simulink model "SimulinkPacer"  (R2022a)
settings: Solver=FixedStepAuto  StartTime=0.0  StopTime=10.0  FixedStep=1e-3  RelTol=1e-3  EnableMultiTasking=on
undefined symbols (not defined in the file): D0, D1, D10, D11, D12, D13, D2, D3, D4, D5, D6, D7, D8, D9, PTA0, PTA1, PTA2, PTB23, PTB9, PTC16, PTC17, PTC2, PTC3, PTC4, PTD0, PTD1, PTD2, PTD3
libraries: frdmk64flib x17
settings Model: ExtModeTrigDuration=5  Creator=sabri  LastModifiedBy=Tim
settings SolverCC: AlgebraicLoopSolver=TrustRegion
settings OptimizationCC: EnhancedBackFolding=on  PassReuseOutputArgsAs=Individual arguments  ZeroExternalMemoryAtStartup=off  ZeroInternalMemoryAtStartup=off  MaxStackSize=64  OptimizeBlockOrder=speed  DifferentSizesBufferReuse=on  OptimizationCustomize=off  EfficientTunableParamExpr=on
settings DebuggingCC: ParameterTunabilityLossMsg=error  UnconnectedInputMsg=warning  UnconnectedOutputMsg=warning  UnconnectedLineMsg=warning  SFMachineParentedDataDiag=warning
settings HardwareCC: ProdBitPerPointer=32  ProdBitPerSizeT=32  ProdBitPerPtrDiffT=32  ProdLargestAtomicInteger=Long  ProdLargestAtomicFloat=Double  ProdWordSize=32  ProdHWDeviceType=ARM Compatible->ARM Cortex
settings SFSimCC: MATLABDynamicMemAlloc=off
settings RTWCC: SystemTargetFile=ert.tlc  HardwareBoard=NXP FRDM-K64F  TLCOptions="-aInlineSetEventsForThisBaseRateFcn=TLC_FALSE -aSuppressMultiTaskScheduler=TLC_FALSE  -aRateBasedStepFcn=0"  TemplateMakefile=ert_default_tmf  Toolchain=GNU Tools for ARM Embedded Processors
settings CodeAppCC: ForceParamTrailComments=on  IgnoreCustomStorageClasses=off  OperatorAnnotations=on  SimulinkDataObjDesc=on  SFDataObjDesc=on  InsertBlockDesc=on

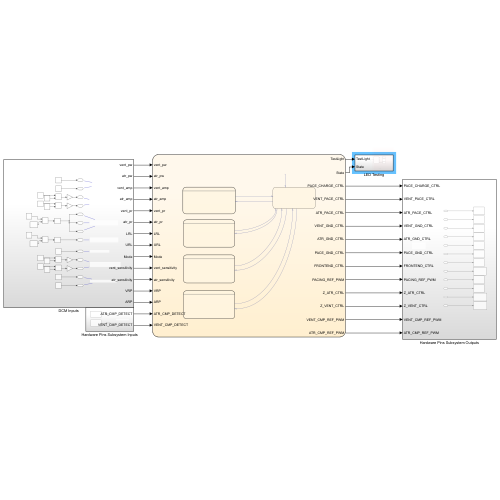
[thumbnail: Simulink's stored preview of the top-level diagram]
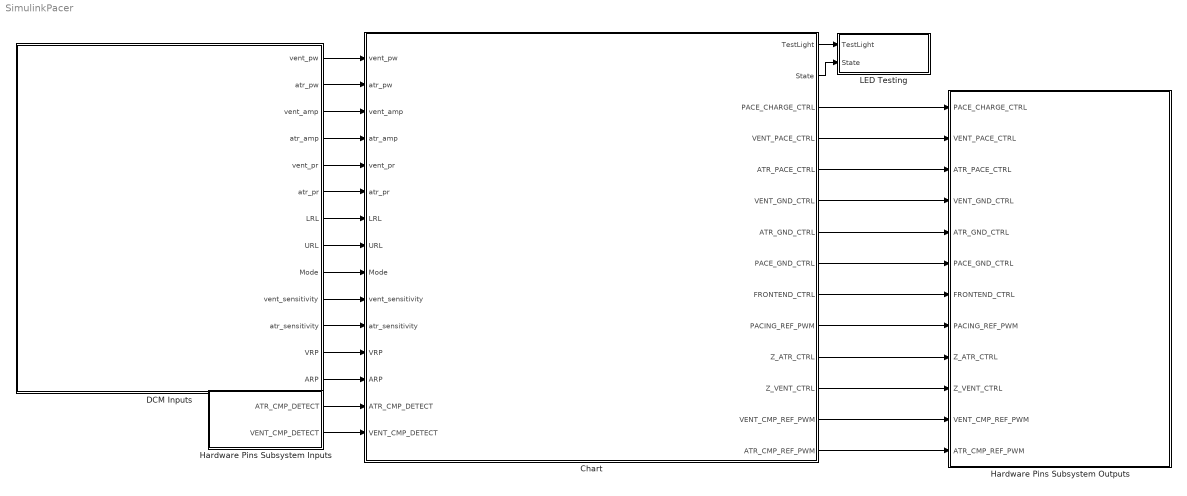
== system SimulinkPacer ==
  Chart : Stateflow chart  TreatAsAtomicUnit=on
      settings: PortSchema="{\"entries\":[{\"content\":{\"sides\":[{\"content\":{\"connectorIds\":[\"In1\",\"In2\",\"In3\",\"In4\",\"In5\",\"In8\",\"In6\",\"In7\",\"In9\",\"In13\",\"In15\",\"In12\",\"In14\",\"In10\",\"In11\"]},\"type\":\"ConnectorPlacement.EquallySpacedRectSide\",\"uuid\":\"c98da620-bdff-4f08-8425-4ebbcd1bf391\"},{\"content\":{\"connectorIds\":[\"Out14\",\"Out1\",\"Out2\",\"Out3\",\"Out4\",\"Out5\",\"Out6\",\"Out7\",\"Out8\",\"Out9\",\"Out10\",\"Out11\",\"Out12\",\"Out13\"],\"side\":\"RIGHT\"},\"type\":\"ConnectorPlacement.EquallySpacedRectSide\",\"uuid\":\"56adc0a6-f124-4dd5-8d25-ce86442aaf81\"},{\"content\":{\"connectorIds\":[],\"side\":\"TOP\"},\"type\":\"ConnectorPlacement.EquallySpacedRectSide\",\"uuid\":\"2a0b7820-84a3-4d69-9bc9-487093068e4c\"}]},\"type\":\"ConnectorPlacement.EquallySpacedConnector\",\"uuid\":\"3fd3921a-48fb-429d-b48c-ef226cae10fe\"}],\"packageUris\":[\"http://schema.mathworks.com/mf0/Connector/R2020b\"],\"version\":\"1.0\"}"
  DCM Inputs : Subsystem
  Hardware Pins Subsystem Inputs : Subsystem
  Hardware Pins Subsystem Outputs : Subsystem
  LED Testing : Subsystem
  wires:
  Chart/2(PACE_CHARGE_CTRL) -> Hardware Pins Subsystem Outputs/1(PACE_CHARGE_CTRL)
  Chart/3(VENT_PACE_CTRL) -> Hardware Pins Subsystem Outputs/2(VENT_PACE_CTRL)
  Chart/4(ATR_PACE_CTRL) -> Hardware Pins Subsystem Outputs/3(ATR_PACE_CTRL)
  Chart/5(VENT_GND_CTRL) -> Hardware Pins Subsystem Outputs/4(VENT_GND_CTRL)
  Chart/6(ATR_GND_CTRL) -> Hardware Pins Subsystem Outputs/5(ATR_GND_CTRL)
  Chart/7(PACE_GND_CTRL) -> Hardware Pins Subsystem Outputs/6(PACE_GND_CTRL)
  Chart/8(FRONTEND_CTRL) -> Hardware Pins Subsystem Outputs/7(FRONTEND_CTRL)
  Chart/9(PACING_REF_PWM) -> Hardware Pins Subsystem Outputs/8(PACING_REF_PWM)
  Chart/10(Z_ATR_CTRL) -> Hardware Pins Subsystem Outputs/9(Z_ATR_CTRL)
  Chart/11(Z_VENT_CTRL) -> Hardware Pins Subsystem Outputs/10(Z_VENT_CTRL)
  DCM Inputs/1(vent_pw) -> Chart/1(vent_pw)
  DCM Inputs/2(atr_pw) -> Chart/2(atr_pw)
  DCM Inputs/3(vent_amp) -> Chart/3(vent_amp)
  DCM Inputs/4(atr_amp) -> Chart/4(atr_amp)
  DCM Inputs/5(vent_pr) -> Chart/5(vent_pr)
  DCM Inputs/6(atr_pr) -> Chart/8(atr_pr)
  DCM Inputs/9(Mode) -> Chart/9(Mode)
  Hardware Pins Subsystem Inputs/2(VENT_CMP_DETECT) -> Chart/11(VENT_CMP_DETECT)
  Hardware Pins Subsystem Inputs/1(ATR_CMP_DETECT) -> Chart/10(ATR_CMP_DETECT)
  DCM Inputs/7(LRL) -> Chart/6(LRL)
  DCM Inputs/8(URL) -> Chart/7(URL)
  DCM Inputs/12(VRP) -> Chart/12(VRP)
  DCM Inputs/13(ARP) -> Chart/14(ARP)
  DCM Inputs/10(vent_sensitivity) -> Chart/13(vent_sensitivity)
  DCM Inputs/11(atr_sensitivity) -> Chart/15(atr_sensitivity)
  Chart/12(VENT_CMP_REF_PWM) -> Hardware Pins Subsystem Outputs/11(VENT_CMP_REF_PWM)
  Chart/13(ATR_CMP_REF_PWM) -> Hardware Pins Subsystem Outputs/12(ATR_CMP_REF_PWM)
  Chart/1(State) -> LED Testing/2(State)
  Chart/14(TestLight) -> LED Testing/1(TestLight)

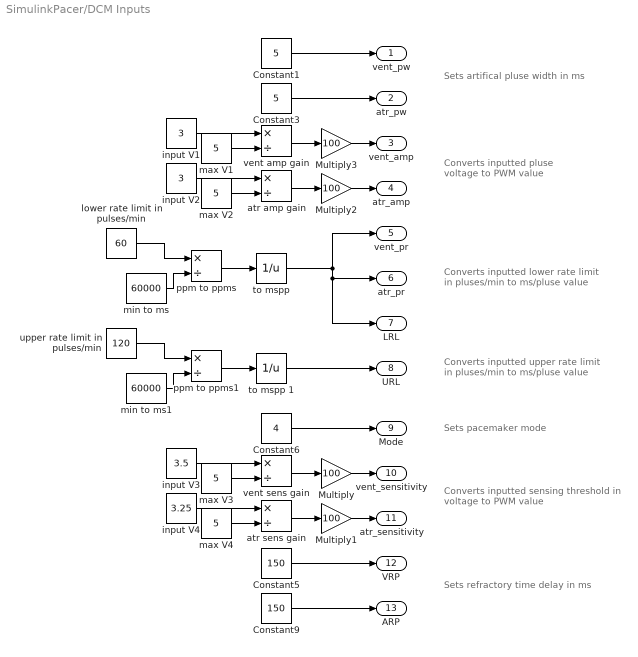
== system SimulinkPacer/DCM Inputs ==
  note: Converts inputted pluse
      | voltage to PWM value
  note: Converts inputted lower rate limit
      | in pluses/min to ms/pluse value
  note: Converts inputted upper rate limit
      | in pluses/min to ms/pluse value
  note: Converts inputted sensing threshold
      | in voltage to PWM value
  note: Sets artifical pluse width in ms
  note: Sets pacemaker mode
  note: Sets refractory time delay in ms
  Constant1 : Constant  Value=5
  Constant3 : Constant  Value=5
  Constant5 : Constant  Value=150
  Constant6 : Constant  Value=4
  Constant9 : Constant  Value=150
  Multiply{,1..3} (4 alike) : Gain  Gain=100
  atr amp gain : Product  Inputs=*/
  atr sens gain : Product  Inputs=*/
  input V1 : Constant  Value=3
  input V2 : Constant  Value=3
  input V3 : Constant  Value=3.5
  input V4 : Constant  Value=3.25
  lower rate limit in pulses/min : Constant  Value=60
  max V{1..4} (4 alike) : Constant  Value=5
  min to ms : Constant  Value=60000
  min to ms1 : Constant  Value=60000
  ppm to ppms : Product  Inputs=*/
  ppm to ppms1 : Product  Inputs=*/
  "to mspp " : Math  Operator=reciprocal
  to mspp 1 : Math  Operator=reciprocal
  upper rate limit in pulses/min : Constant  Value=120
  vent amp gain : Product  Inputs=*/
  vent sens gain : Product  Inputs=*/
  vent_pw : Outport
  atr_pw : Outport  Port=2
  vent_amp : Outport  Port=3
  atr_amp : Outport  Port=4
  vent_pr : Outport  Port=5
  atr_pr : Outport  Port=6
  LRL : Outport  Port=7
  URL : Outport  Port=8
  Mode : Outport  Port=9
  vent_sensitivity : Outport  Port=10
  atr_sensitivity : Outport  Port=11
  VRP : Outport  Port=12
  ARP : Outport  Port=13
  wires:
  Constant6/1 -> Mode/1
  ppm to ppms/1 -> "to mspp "/1
  min to ms/1 -> ppm to ppms/2
  "to mspp "/1 -> vent_pr/1, LRL/1, atr_pr/1
  lower rate limit in pulses/min/1 -> ppm to ppms/1
  Constant3/1 -> atr_pw/1
  Constant1/1 -> vent_pw/1
  ppm to ppms1/1 -> to mspp 1/1
  min to ms1/1 -> ppm to ppms1/2
  to mspp 1/1 -> URL/1
  upper rate limit in pulses/min/1 -> ppm to ppms1/1
  Constant5/1 -> VRP/1
  Constant9/1 -> ARP/1
  max V2/1 -> atr amp gain/2
  input V2/1 -> atr amp gain/1
  input V1/1 -> vent amp gain/1
  max V1/1 -> vent amp gain/2
  input V3/1 -> vent sens gain/1
  max V3/1 -> vent sens gain/2
  max V4/1 -> atr sens gain/2
  input V4/1 -> atr sens gain/1
  Multiply/1 -> vent_sensitivity/1
  Multiply1/1 -> atr_sensitivity/1
  vent sens gain/1 -> Multiply/1
  atr sens gain/1 -> Multiply1/1
  Multiply2/1 -> atr_amp/1
  Multiply3/1 -> vent_amp/1
  vent amp gain/1 -> Multiply3/1
  atr amp gain/1 -> Multiply2/1

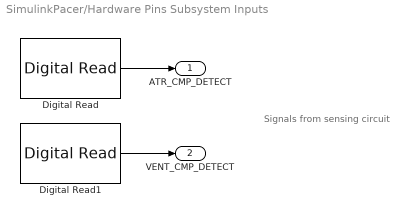
== system SimulinkPacer/Hardware Pins Subsystem Inputs ==
  note: Signals from sensing circuit
  Digital Read : frdmk64flib/Digital Read  Whichpin=PTC16 (D0)  SampleTime=-1
  Digital Read1 : frdmk64flib/Digital Read  Whichpin=PTC17 (D1)  SampleTime=-1
  ATR_CMP_DETECT : Outport
  VENT_CMP_DETECT : Outport  Port=2
  wires:
  Digital Read1/1 -> VENT_CMP_DETECT/1
  Digital Read/1 -> ATR_CMP_DETECT/1

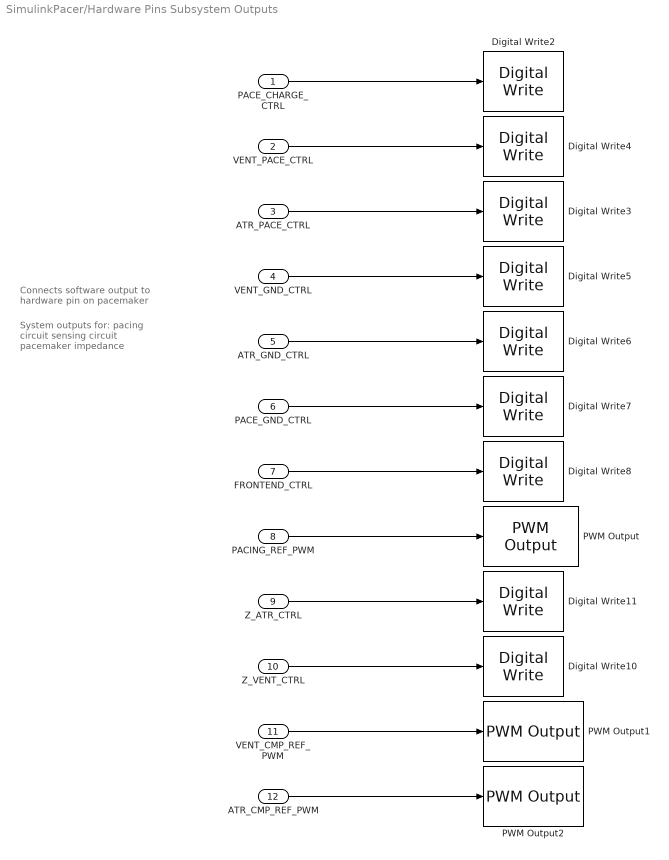
== system SimulinkPacer/Hardware Pins Subsystem Outputs ==
  note: System outputs for:
      | pacing circuit
      | sensing circuit
      | pacemaker impedance
  note: Connects software output to
      | hardware pin on pacemaker
  PACE_CHARGE_CTRL : Inport
  VENT_PACE_CTRL : Inport  Port=2
  ATR_PACE_CTRL : Inport  Port=3
  VENT_GND_CTRL : Inport  Port=4
  ATR_GND_CTRL : Inport  Port=5
  PACE_GND_CTRL : Inport  Port=6
  FRONTEND_CTRL : Inport  Port=7
  PACING_REF_PWM : Inport  Port=8
  Z_ATR_CTRL : Inport  Port=9
  Z_VENT_CTRL : Inport  Port=10
  VENT_CMP_REF_PWM : Inport  Port=11
  ATR_CMP_REF_PWM : Inport  Port=12
  Digital Write10 : frdmk64flib/Digital Write  Whichpin=PTC3 (D7)
  Digital Write11 : frdmk64flib/Digital Write  Whichpin=PTB23 (D4)
  Digital Write2 : frdmk64flib/Digital Write  Whichpin=PTB9 (D2)
  Digital Write3 : frdmk64flib/Digital Write  Whichpin=PTA0 (D8)
  Digital Write4 : frdmk64flib/Digital Write  Whichpin=PTC4 (D9)
  Digital Write5 : frdmk64flib/Digital Write  Whichpin=PTD3 (D12)
  Digital Write6 : frdmk64flib/Digital Write  Whichpin=PTD2 (D11)
  Digital Write7 : frdmk64flib/Digital Write  Whichpin=PTD0 (D10)
  Digital Write8 : frdmk64flib/Digital Write  Whichpin=PTD1 (D13)
  PWM Output : frdmk64flib/PWM Output  Whichpin=PTA2 (D5)  InitialFrequency=2000  InitialDutyCycle=0
  PWM Output1 : frdmk64flib/PWM Output  Whichpin=PTA1 (D3)  InitialFrequency=2000  InitialDutyCycle=0
  PWM Output2 : frdmk64flib/PWM Output  Whichpin=PTC2 (D6)  InitialFrequency=2000  InitialDutyCycle=0
  wires:
  PACE_CHARGE_CTRL/1 -> Digital Write2/1
  VENT_PACE_CTRL/1 -> Digital Write4/1
  ATR_PACE_CTRL/1 -> Digital Write3/1
  VENT_GND_CTRL/1 -> Digital Write5/1
  ATR_GND_CTRL/1 -> Digital Write6/1
  PACE_GND_CTRL/1 -> Digital Write7/1
  FRONTEND_CTRL/1 -> Digital Write8/1
  PACING_REF_PWM/1 -> PWM Output/1
  Z_ATR_CTRL/1 -> Digital Write11/1
  Z_VENT_CTRL/1 -> Digital Write10/1
  VENT_CMP_REF_PWM/1 -> PWM Output1/1
  ATR_CMP_REF_PWM/1 -> PWM Output2/1

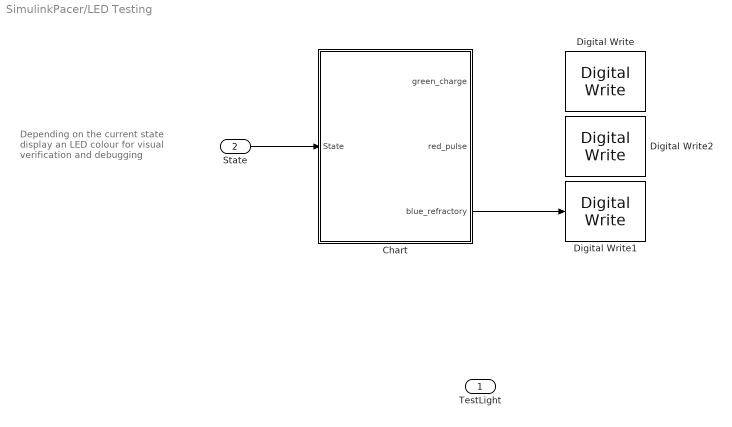
== system SimulinkPacer/LED Testing ==
  note: Depending on the current state
      | display an LED colour for visual
      | verification and debugging
  TestLight : Inport
  State : Inport  Port=2
  Chart : Stateflow chart  TreatAsAtomicUnit=on
  Digital Write : frdmk64flib/Digital Write  Whichpin=GREEN_LED
  Digital Write1 : frdmk64flib/Digital Write  Whichpin=BLUE_LED
  Digital Write2 : frdmk64flib/Digital Write  Whichpin=RED_LED
  wires:
  State/1 -> Chart/1(State)
  Chart/3(blue_refractory) -> Digital Write1/1

== stateflow chart SimulinkPacer/LED Testing/Chart ==
  state Charge_Setting
    entry:
    green_charge = 1
    red_pulse = 0
    blue_refractory = 0
  state Pulse_Setting
    entry:
    green_charge = 0
    red_pulse = 1
    blue_refractory = 0
  state Start
  state Refractory_Setting
    entry:
    green_charge = 0
    red_pulse = 0
    blue_refractory = 1
  Start -> Charge_Setting [order 3] : [State == 0]
  Charge_Setting -> Start
  (default) -> Start
  Start -> Pulse_Setting [order 1] : [State == 1]
  Pulse_Setting -> Start
  Start -> Refractory_Setting [order 2] : [State == 2]
  Refractory_Setting -> Start
  data: green_charge output; red_pulse output; State input; blue_refractory output

== stateflow chart SimulinkPacer/Chart ==
  state VOO
    state VOO_Pacing
      % Paces heart
      % Configures pacing circuit for charging
      % Disables sensing circuit
      % Configures pacemaker impedance
      entry:
      State = 1
      PACE_CHARGE_CTRL = 0
      PACE_GND_CTRL = 1
      ATR_PACE_CTRL = 0
      ATR_GND_CTRL = 0
      Z_ATR_CTRL = 0
      Z_VENT_CTRL = 0
      VENT_GND_CTRL = 0
      VENT_PACE_CTRL = 1
      FRONTEND_CTRL = 0
      PACING_REF_PWM = vent_amp
    state VOO_Charging
      % Charges pacemaker
      % Configures pacing circuit for charging
      % Disables sensing circuit
      % Configures pacemaker impedance
      entry:
      State = 0
      PACE_GND_CTRL = 1
      VENT_PACE_CTRL = 0
      Z_ATR_CTRL = 0
      Z_VENT_CTRL = 0
      ATR_GND_CTRL = 0
      VENT_GND_CTRL = 1
      ATR_PACE_CTRL = 0
      PACING_REF_PWM = vent_amp
      PACE_CHARGE_CTRL = 1
      FRONTEND_CTRL = 0
    VOO_Pacing -> VOO_Charging : [after(vent_pw, msec)]
        | % time delay after pacing
    (default) -> VOO_Charging
    VOO_Charging -> VOO_Pacing : [after(vent_pr - vent_pw, msec)]
        | % time delay after charging pacemaker
  state ModeSelect
    % Determines the pacemaker mode
    % Mode 1 = VOO
    % Mode 2 = AOO
    % Mode 3 = VVI
    % Mode 4 = AAI
  state AOO
    state AOO_Pacing
      % Paces heart
      % Configures pacing circuit for pacing
      % Disables sensing circuit
      % Configures pacemaker impedance
      entry:
      State = 1
      PACE_CHARGE_CTRL = 0
      PACE_GND_CTRL = 1
      ATR_PACE_CTRL = 1
      ATR_GND_CTRL = 0
      Z_ATR_CTRL = 0
      Z_VENT_CTRL = 0
      VENT_GND_CTRL = 0
      VENT_PACE_CTRL = 0
      FRONTEND_CTRL = 0
      PACING_REF_PWM = atr_amp
    state AOO_Charging
      % Charges pacemaker
      % Configures pacing circuit for charging
      % Disables sensing circuit
      % Configures pacemaker impedance
      entry:
      State = 0
      PACE_GND_CTRL = 1
      VENT_PACE_CTRL = 0
      Z_ATR_CTRL = 0
      Z_VENT_CTRL = 0
      ATR_GND_CTRL = 1
      VENT_GND_CTRL = 0
      ATR_PACE_CTRL = 0
      PACING_REF_PWM = atr_amp
      PACE_CHARGE_CTRL = 1
      FRONTEND_CTRL = 0
    AOO_Pacing -> AOO_Charging : [after(atr_pw, msec)]
        | % time delay after pacing
    (default) -> AOO_Charging
    AOO_Charging -> AOO_Pacing : [after(atr_pr - atr_pw, msec)]
        | % time delay after charing pacemaker
  state VVI
    state VVI_Refractory
      % Waits specified time before sensing
      % Configures pacing circuit for charging
      % Ignores sensing signals
      % Configures pacemaker impedance
      entry:
      artificial_pace = 0
      State = 2
      %FRONTEND_CTRL = 0 % not sensing caused errors
      VENT_CMP_REF_PWM = vent_sensitivity
      PACE_GND_CTRL = 1
      VENT_PACE_CTRL = 0
      Z_ATR_CTRL = 0
      Z_VENT_CTRL = 0
      ATR_GND_CTRL = 0
      VENT_GND_CTRL = 1
      ATR_PACE_CTRL = 0
      PACING_REF_PWM = vent_amp
      PACE_CHARGE_CTRL = 1
    state VVI_Pacing
      % Paces heart
      % Configures pacing circuit for pacing
      % Ignores sensing signals
      % Configures pacemaker impedance
      entry:
      State = 1
      TestLight = 0
      FRONTEND_CTRL = 1 % sensing
      VENT_CMP_REF_PWM = vent_sensitivity
      PACE_CHARGE_CTRL = 0
      PACE_GND_CTRL = 1
      ATR_PACE_CTRL = 0
      ATR_GND_CTRL = 0
      Z_ATR_CTRL = 0
      Z_VENT_CTRL = 0
      VENT_GND_CTRL = 0
      VENT_PACE_CTRL = 1
      PACING_REF_PWM = vent_amp
    state VVI_Charging
      % Charges pacemaker
      % Sensing for natural pluse
      % Configures pacing circuit for charging
      % Configures pacemaker impedance
      entry:
      State = 0
      TestLight = 0
      FRONTEND_CTRL = 1 % sensing
      VENT_CMP_REF_PWM = vent_sensitivity
      PACE_GND_CTRL = 1
      VENT_PACE_CTRL = 0
      Z_ATR_CTRL = 0
      Z_VENT_CTRL = 0
      ATR_GND_CTRL = 0
      VENT_GND_CTRL = 1
      ATR_PACE_CTRL = 0
      PACING_REF_PWM = vent_amp
      PACE_CHARGE_CTRL = 1
    VVI_Charging -> VVI_Refractory [order 1] : [VENT_CMP_DETECT == 1]
        | % pulse detected, do not pulse artificially
    VVI_Pacing -> VVI_Refractory : [after(vent_pw, msec)]
        | {artificial_pace = 1}
        | % time delay for pacing
    VVI_Charging -> VVI_Pacing [order 2] : [after(LRL - vent_pw*artificial_pace - VRP, msec)]
        | % no pulse detected in allowable
        | % time from LRL, pulse artificially
    (default) -> VVI_Charging
    VVI_Refractory -> VVI_Charging : [after(VRP, msec)]
        | % time delay for refractory period
  state AAI
    state AAI_Refractory
      % Waits specified time before sensing
      % Configures pacing circuit for charging
      % Ignores sensing signals
      % Configures pacemaker impedance
      entry:
      artificial_pace = 0
      State = 2
      %FRONTEND_CTRL = 0 % not sensing caused errors
      ATR_CMP_REF_PWM = atr_sensitivity
      PACE_GND_CTRL = 1
      VENT_PACE_CTRL = 0
      Z_ATR_CTRL = 0
      Z_VENT_CTRL = 0
      ATR_GND_CTRL = 1
      VENT_GND_CTRL = 0
      ATR_PACE_CTRL = 0
      PACING_REF_PWM = atr_amp
      PACE_CHARGE_CTRL = 1
    state AAI_Pacing
      % Paces heart
      % Configures pacing circuit for pacing
      % Ignores sensing signals
      % Configures pacemaker impedance
      entry:
      State = 1
      FRONTEND_CTRL = 1 % sensing
      ATR_CMP_REF_PWM = atr_sensitivity
      PACE_CHARGE_CTRL = 0
      PACE_GND_CTRL = 1
      ATR_PACE_CTRL = 1
      ATR_GND_CTRL = 0
      Z_ATR_CTRL = 0
      Z_VENT_CTRL = 0
      VENT_GND_CTRL = 0
      VENT_PACE_CTRL = 0
      PACING_REF_PWM = atr_amp
    state AAI_Charging
      % Charges pacemaker
      % Sensing for natural pluse
      % Configures pacing circuit for charging
      % Configures pacemaker impedance
      entry:
      State = 0
      FRONTEND_CTRL = 1 % sensing
      ATR_CMP_REF_PWM = atr_sensitivity
      PACE_GND_CTRL = 1
      VENT_PACE_CTRL = 0
      Z_ATR_CTRL = 0
      Z_VENT_CTRL = 0
      ATR_GND_CTRL = 1
      VENT_GND_CTRL = 0
      ATR_PACE_CTRL = 0
      PACING_REF_PWM = atr_amp
      PACE_CHARGE_CTRL = 1
    AAI_Charging -> AAI_Refractory [order 1] : [ATR_CMP_DETECT == 1]
        | % pulse detected, do not pulse artificially
    AAI_Pacing -> AAI_Refractory : [after(atr_pw, msec)]
        | {artificial_pace = 1}
        | % time delay pacing
    (default) -> AAI_Charging
    AAI_Charging -> AAI_Pacing [order 2] : [after(LRL - atr_pw*artificial_pace - ARP, msec)]
        | % no pulse detected in allowable
        | % time from LRL, pulse artificially
    AAI_Refractory -> AAI_Charging : [after(ARP, msec)]
        | % time delay in refractory period
  (default) -> ModeSelect
  VOO -> ModeSelect : [Mode ~= 1]
  ModeSelect -> VOO [order 2] : [Mode == 1]
  AAI -> ModeSelect : [Mode ~= 4]
  VVI -> ModeSelect : [Mode ~= 3]
  ModeSelect -> VVI [order 4] : [Mode == 3]
  ModeSelect -> AAI [order 1] : [Mode == 4]
  AOO -> ModeSelect : [Mode ~= 2]
  ModeSelect -> AOO [order 3] : [Mode == 2]
  data: vent_pw input; atr_pw input; vent_amp input; atr_amp input; vent_pr input; LRL input; URL input; atr_pr input; State output double =0; PACE_CHARGE_CTRL output; VENT_PACE_CTRL output; ATR_PACE_CTRL output; VENT_GND_CTRL output; ATR_GND_CTRL output; PACE_GND_CTRL output; FRONTEND_CTRL output; PACING_REF_PWM output; Z_ATR_CTRL output; Z_VENT_CTRL output; Mode input; ATR_CMP_DETECT input; VENT_CMP_DETECT input; VRP input; VENT_CMP_REF_PWM output; ATR_CMP_REF_PWM output; vent_sensitivity input double; ARP input; atr_sensitivity input double; prev_pace local; TestLight output; natural_pace local; artificial_pace local
